simulink model "Counter_Stateflow"  (R2021a)
settings: Solver=FixedStepDiscrete  StartTime=0.0  StopTime=20  RelTol=1e-3  EnableMultiTasking=on
settings Model: Creator=omar  LastModifiedBy=omar
settings DataIOCC: ReturnWorkspaceOutputs=off
settings OptimizationCC: DefaultParameterBehavior=Inlined  InlineInvariantSignals=on  EnableMemcpy=off  LifeSpan=1  EfficientTunableParamExpr=on
settings DebuggingCC: UnderspecifiedInitializationDetection=Classic  MergeDetectMultiDrivingBlocksExec=none  SFMachineParentedDataDiag=warning  ArithmeticOperatorsInVariantConditions=warning
settings ModelReferenceCC: PropagateSignalLabelsOutOfModel=off
settings SFSimCC: MATLABDynamicMemAlloc=off  CustomCodeUndefinedFunction=UseInterfaceOnly
settings RTWCC: SystemTargetFile=ert.tlc  GenCodeOnly=on  TemplateMakefile=ert_default_tmf  GenerateReport=on  IncludeHyperlinkInReport=on  LaunchReport=on  GenerateTraceInfo=on  GenerateTraceReport=on  GenerateTraceReportSl=on  GenerateTraceReportSf=on  GenerateTraceReportEml=on
settings CodeAppCC: ForceParamTrailComments=on  IgnoreCustomStorageClasses=off  OperatorAnnotations=on  SimulinkDataObjDesc=on  SFDataObjDesc=on  MATLABFcnDesc=on  InsertBlockDesc=on  StateflowObjectComments=on  MATLABSourceComments=on
settings ERTTargetCC: MultiwordLength=2048  GenerateSampleERTMain=on  InlinedParameterPlacement=NonHierarchical  ERTCustomFileTemplate=example_file_process.tlc

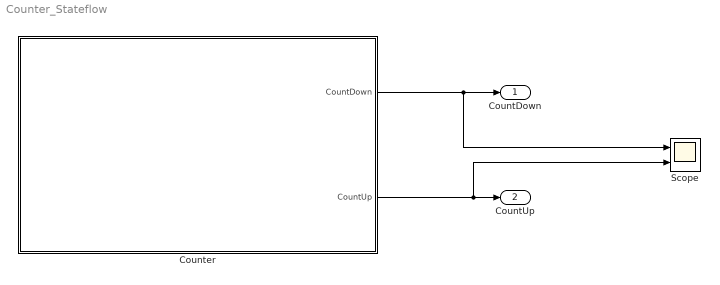
== system Counter_Stateflow ==
  Counter : Stateflow chart  TreatAsAtomicUnit=on
      settings: RTWSystemCode=Reusable function  RTWFcnNameOpts=Use subsystem name  RTWFileNameOpts=Use subsystem name
  Scope : Scope  NumInputPorts=2
  CountDown : Outport
  CountUp : Outport  Port=2
  wires:
  Counter/1(CountDown) -> Scope/1, CountDown/1
  Counter/2(CountUp) -> Scope/2, CountUp/1

== stateflow chart Counter_Stateflow/Counter ==
  state CountUp_And_Down_Modifier
    entry:
    CountUp = CountUp + 1;
    CountDown = CountDown - 1;
  state Reset
    entry:
    CountUp = 0;
    CountDown = 10;
  (default) -> CountUp_And_Down_Modifier
  CountUp_And_Down_Modifier -> CountUp_And_Down_Modifier [order 2] : after(1,tick)
  Reset -> CountUp_And_Down_Modifier
  CountUp_And_Down_Modifier -> Reset [order 1] : [CountUp == 10]
  data: CountDown output =11; CountUp output =-1
